simulink model "JCBM_S"  (R2020b)
settings: Solver=ode45  StartTime=0.0  StopTime=t_sim  MaxStep=1e-3  RelTol=1e-3  EnableMultiTasking=on
model workspace (MAT data in the model file):
  t_sim = 1
values from neighbouring files (symbols this model uses):
  Cfi = Cfin; clear Cfin    [JCBM_M.m]
  Jm = 10*J    (= 5)    [JCBM_M.m]
  Ka = 1/Ra    (= 1.41843971631)    [JCBM_M.m]
  Mz = Mn    (= 339)    [JCBM_M.m]
  Ta = La/Ra    (= 0.0128368794326)    [JCBM_M.m]
  Ua = Un    (= 400)    [JCBM_M.m]
settings Model: Creator=student  LastModifiedBy=andre
settings DataIOCC: LimitDataPoints=on  SaveFormat=Array  ReturnWorkspaceOutputs=off
settings OptimizationCC: LifeSpan=inf
settings DebuggingCC: UnderspecifiedInitializationDetection=Classic  MergeDetectMultiDrivingBlocksExec=none  SolverPrmCheckMsg=warning  SFUnexpectedBacktrackingDiag=warning  SFNoUnconditionalDefaultTransitionDiag=warning  SFExecutionAtInitializationDiag=none  ArithmeticOperatorsInVariantConditions=warning
settings HardwareCC: ProdBitPerPointer=32  ProdBitPerSizeT=32  ProdBitPerPtrDiffT=32  ProdLargestAtomicFloat=None  ProdIntDivRoundTo=Undefined  ProdEndianess=Unspecified  ProdWordSize=32  ProdHWDeviceType=32-bit Generic
settings ModelReferenceCC: PropagateSignalLabelsOutOfModel=off
settings SFSimCC: SimUseLocalCustomCode=off  CustomCodeUndefinedFunction=UseInterfaceOnly
settings RTWCC: RTWUseLocalCustomCode=off
settings CodeAppCC: StateflowObjectComments=on
settings GRTTargetCC: TargetLangStandard=C89/C90 (ANSI)
settings ConfigComp: CovMetricSettings=dw  CovSaveCumulativeToWorkspaceVar=on  CovSaveSingleToWorkspaceVar=on  CovExternalEMLEnable=off

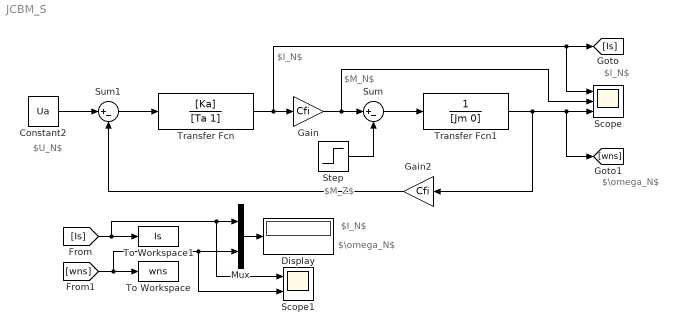
== system JCBM_S ==
  note: $I_N$
  note: $\omega_N$
  note: $U_N$
  note: $M_Z$
  note: $M_N$
  note: $I_N$
  note: $\omega_N$
  note: $I_N$
  Constant2 : Constant  Value=Ua
  Display : Display
  Gain : Gain  Gain=Cfi
  Gain2 : Gain  Gain=Cfi
  Mux : Mux  Inputs=2
  Scope : Scope  NumInputPorts=3
  Scope1 : Scope  NumInputPorts=2
  Step : Step  Time=t_sim/2  After=Mz  SampleTime=0
  Sum : Sum  Inputs=|+-
  Sum1 : Sum  Inputs=|+-
  To Workspace : ToWorkspace  VariableName=wns  SaveFormat=Timeseries  SampleTime=-1
  To Workspace1 : ToWorkspace  VariableName=Is  SaveFormat=Timeseries  SampleTime=-1
  Transfer Fcn : TransferFcn  Numerator=[Ka]  Denominator=[Ta 1]
  Transfer Fcn1 : TransferFcn  Denominator=[Jm 0]
  wires:
  Sum1/1 -> Transfer Fcn/1
  Transfer Fcn/1 -> [Is], Scope/1, Gain/1
  Gain/1 -> Scope/2, Sum/1
  Transfer Fcn1/1 -> Scope/3, [wns], Gain2/1
  Sum/1 -> Transfer Fcn1/1
  Gain2/1 -> Sum1/2
  Step/1 -> Sum/2
  Constant2/1 -> Sum1/1
  [Is] -> To Workspace1/1, Scope1/1, Mux/1
  [wns] -> To Workspace/1, Scope1/2, Mux/2
  Mux/1 -> Display/1
